simulink library "dlbsBlockSgd"  (R2025b)
settings: Solver=VariableStepAuto  StartTime=0.0  StopTime=10.0  RelTol=1e-3
libraries: dlbsBlockExtractGradientGF x1
settings Model: Creator=lt6037  LastModifiedBy=lt6037

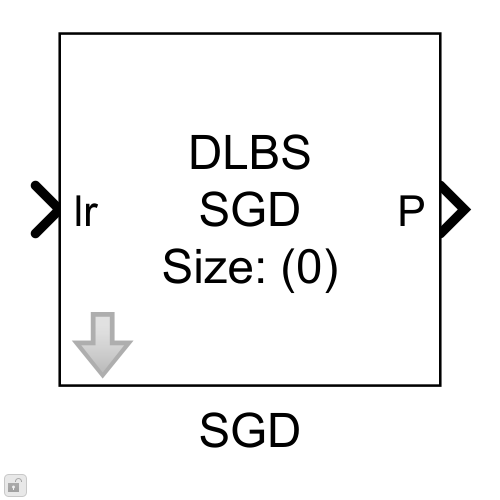
[thumbnail: Simulink's stored preview of the top-level diagram]
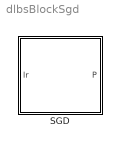
== system dlbsBlockSgd ==
  SGD : Subsystem  mask{init=randn(1,1)}
      mask prompts: init "Initial Values"
      mask help:
      | Updates parameters using stochastic gradient descent.
      | Learnable parameters are owned by the optimizer. The output parameter tensor P is created and sized according to the init parameter.
      mask Help: web("dlbsHelpBlockSgd.html")
      mask Display:
      | try
      |     maskWs = Simulink.Mask.get(gcb).getWorkspace();
      |     sizeArray = size(maskWs.get("init"));
      | catch
      |     sizeArray = 0;
      | end
      | 
      | sizeString="(";
      | 
      | for k = 1:length(sizeArray)
      |     sizeString = sizeString+num2str(sizeArray(k));
      |     if k < length(sizeArray)
      |         sizeString = sizeString + ",";
      |     end
      | end
      | sizeString = sizeString + ")";
      | 
      | 
      | fprintf("DLBS\nSGD\nSize: %s",sizeString)

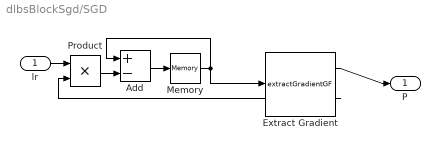
== system dlbsBlockSgd/SGD ==
  lr : Inport
  Add : Sum  Inputs=+-
  Extract Gradient : dlbsBlockExtractGradientGF/extractGradientGF
  Memory : Memory  InitialCondition=init  InheritSampleTime=on
  Product : Product
  P : Outport
  wires:
  Memory/1 -> Extract Gradient/1, Add/1
  lr/1 -> Product/1
  Add/1 -> Memory/1
  Extract Gradient/2 -> Product/2
  Product/1 -> Add/2
  Extract Gradient/1 -> P/1
